simulink model "Motor_moddel"  (R2026a)
settings: Solver=VariableStepAuto
values from neighbouring files (symbols this model uses):
  B = 0.15    [Motor_model_param.m]
  gear = 9.68    [Motor_model_param.m]
  Kp = 0.05    [Motor_model_param.m]    (also in Vel_controller.m = 0.136458313659)
  wrad = 0.03    [Motor_model_param.m]
settings Model: Creator=mariu  LastModifiedBy=mariu

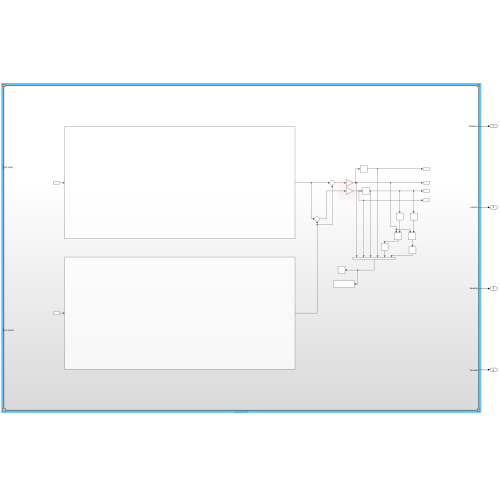
[thumbnail: Simulink's stored preview of the top-level diagram]
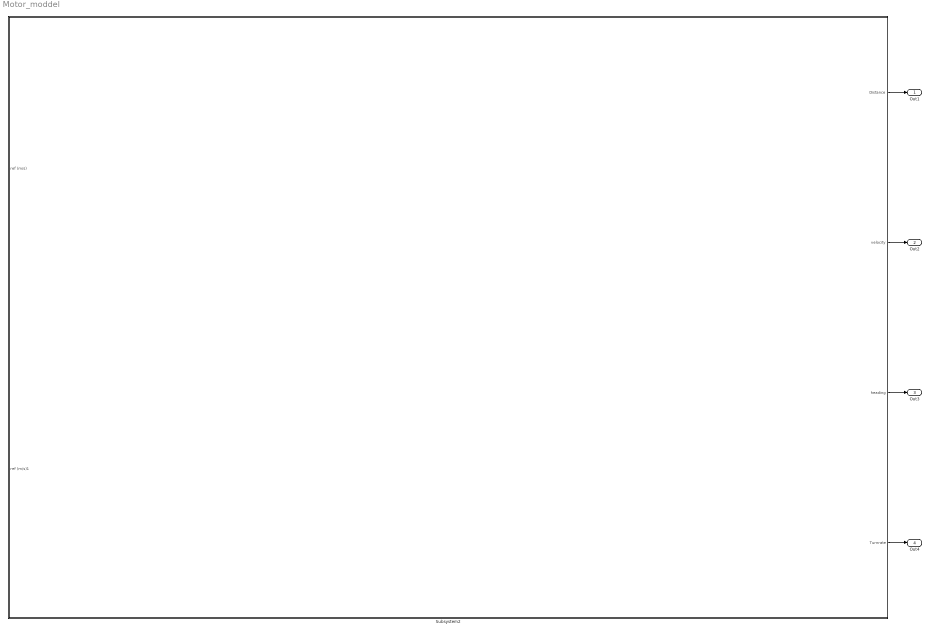
== system Motor_moddel ==
  Subsystem2 : Subsystem
  Out1 : Outport
  Out2 : Outport  Port=2
  Out3 : Outport  Port=3
  Out4 : Outport  Port=4
  wires:
  Subsystem2/1(Distance) -> Out1/1
  Subsystem2/2(velocity) -> Out2/1
  Subsystem2/3(heading) -> Out3/1
  Subsystem2/4(Turnrate) -> Out4/1

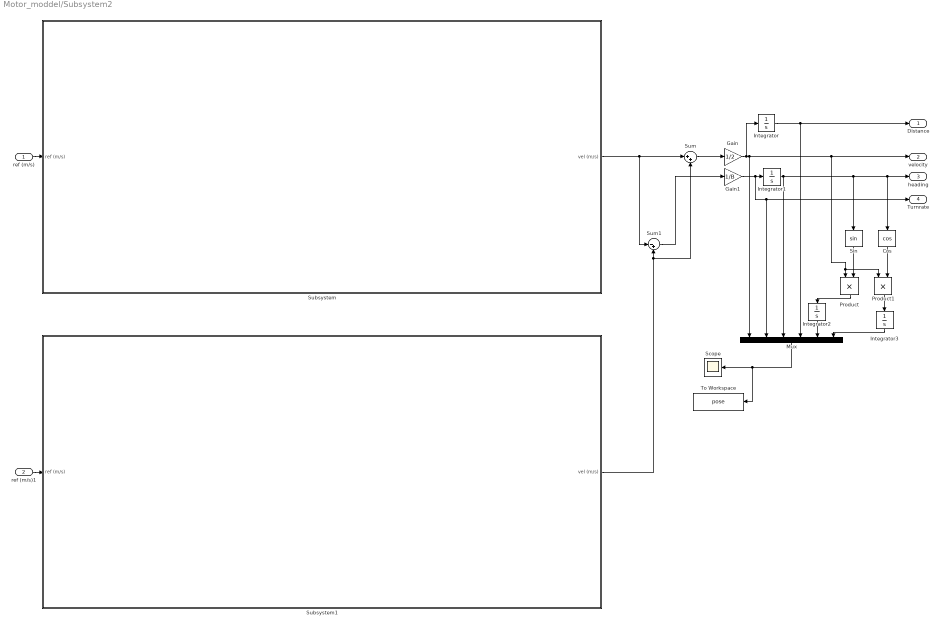
== system Motor_moddel/Subsystem2 ==
  ref (m/s) : Inport
  ref (m/s)1 : Inport  Port=2
  Cos : Trigonometry  Operator=cos
  Gain : Gain  Gain=1/2
  Gain1 : Gain  Gain=1/B
  Integrator{,1..3} (4 alike) : Integrator
  Mux : Mux  Inputs=6
  Product : Product
  Product1 : Product
  Scope : Scope
  Sin : Trigonometry
  Subsystem : Subsystem
  Subsystem1 : Subsystem
  Sum : Sum  Inputs=|++
  Sum1 : Sum  Inputs=|-+
  To Workspace : ToWorkspace  VariableName=pose  SaveFormat=Timeseries  SampleTime=-1
  Distance : Outport
  velocity : Outport  Port=2
  heading : Outport  Port=3
  Turnrate : Outport  Port=4
  wires:
  Integrator1/1 -> Mux/3, Sin/1, heading/1, Cos/1
  Subsystem/1(vel (m/s)) -> Sum1/1, Sum/1
  Gain/1 -> Mux/1, velocity/1, Product1/1, Product/1, Integrator/1
  Gain1/1 -> Turnrate/1, Mux/2, Integrator1/1
  Integrator3/1 -> Mux/6
  Subsystem1/1(vel (m/s)) -> Sum/2, Sum1/2
  Product1/1 -> Integrator3/1
  Mux/1 -> To Workspace/1, Scope/1
  Sum/1 -> Gain/1
  Integrator/1 -> Distance/1, Mux/4
  Sin/1 -> Product/2
  Integrator2/1 -> Mux/5
  Sum1/1 -> Gain1/1
  Cos/1 -> Product1/2
  Product/1 -> Integrator2/1
  ref (m/s)1/1 -> Subsystem1/1(ref (m/s))
  ref (m/s)/1 -> Subsystem/1(ref (m/s))

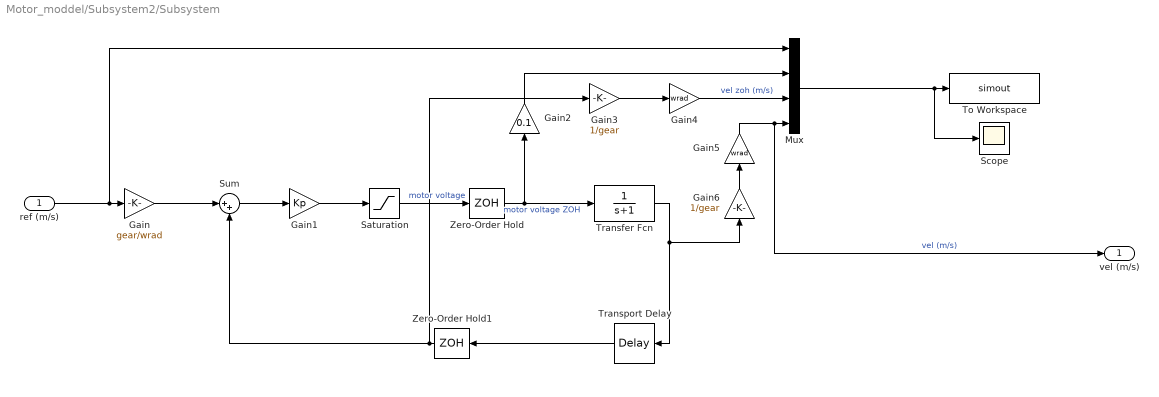
== system Motor_moddel/Subsystem2/Subsystem ==
  ref (m/s) : Inport
  Gain : Gain  Gain=gear/wrad
  Gain1 : Gain  Gain=Kp
  Gain2 : Gain  Gain=0.1
  Gain3 : Gain  Gain=1/gear
  Gain4 : Gain  Gain=wrad
  Gain5 : Gain  Gain=wrad
  Gain6 : Gain  Gain=1/gear
  Mux : Mux
  Saturation : Saturate
  Scope : Scope
  Sum : Sum  Inputs=|++
  To Workspace : ToWorkspace  VariableName=simout  SaveFormat=Timeseries  SampleTime=-1
  Transfer Fcn : TransferFcn  Denominator=[1 1]
  Transport Delay : TransportDelay  DelayTime=0.01
  Zero-Order Hold : ZeroOrderHold  SampleTime=-1
  Zero-Order Hold1 : ZeroOrderHold  SampleTime=-1
  vel (m/s) : Outport
  wires:
  Gain5/1 -> vel (m/s)/1, Mux/4  "vel (m/s)"
  Zero-Order Hold/1 -> Transfer Fcn/1, Gain2/1  "motor voltage ZOH"
  Gain4/1 -> Mux/3  "vel zoh (m/s)"
  Mux/1 -> Scope/1, To Workspace/1
  Gain6/1 -> Gain5/1
  Gain1/1 -> Saturation/1
  Gain2/1 -> Mux/2
  Transfer Fcn/1 -> Gain6/1, Transport Delay/1
  Gain3/1 -> Gain4/1
  Zero-Order Hold1/1 -> Gain3/1, Sum/2
  ref (m/s)/1 -> Mux/1, Gain/1
  Transport Delay/1 -> Zero-Order Hold1/1
  Saturation/1 -> Zero-Order Hold/1  "motor voltage"
  Gain/1 -> Sum/1
  Sum/1 -> Gain1/1

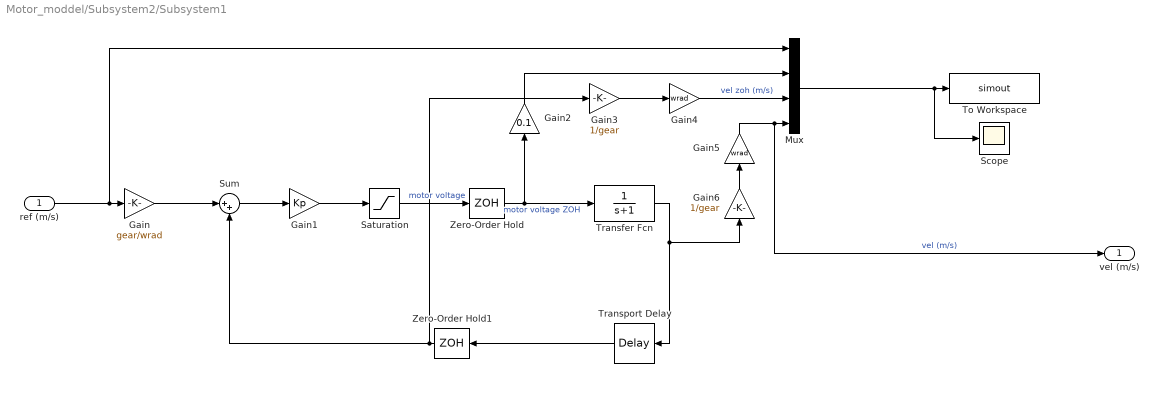
== system Motor_moddel/Subsystem2/Subsystem1 ==
  ref (m/s) : Inport
  Gain : Gain  Gain=gear/wrad
  Gain1 : Gain  Gain=Kp
  Gain2 : Gain  Gain=0.1
  Gain3 : Gain  Gain=1/gear
  Gain4 : Gain  Gain=wrad
  Gain5 : Gain  Gain=wrad
  Gain6 : Gain  Gain=1/gear
  Mux : Mux
  Saturation : Saturate
  Scope : Scope
  Sum : Sum  Inputs=|++
  To Workspace : ToWorkspace  VariableName=simout  SaveFormat=Timeseries  SampleTime=-1
  Transfer Fcn : TransferFcn  Denominator=[1 1]
  Transport Delay : TransportDelay  DelayTime=0.01
  Zero-Order Hold : ZeroOrderHold  SampleTime=-1
  Zero-Order Hold1 : ZeroOrderHold  SampleTime=-1
  vel (m/s) : Outport
  wires:
  Gain5/1 -> vel (m/s)/1, Mux/4  "vel (m/s)"
  Zero-Order Hold/1 -> Transfer Fcn/1, Gain2/1  "motor voltage ZOH"
  Gain4/1 -> Mux/3  "vel zoh (m/s)"
  Mux/1 -> Scope/1, To Workspace/1
  Gain6/1 -> Gain5/1
  Gain1/1 -> Saturation/1
  Gain2/1 -> Mux/2
  Transfer Fcn/1 -> Gain6/1, Transport Delay/1
  Gain3/1 -> Gain4/1
  Zero-Order Hold1/1 -> Gain3/1, Sum/2
  ref (m/s)/1 -> Mux/1, Gain/1
  Transport Delay/1 -> Zero-Order Hold1/1
  Saturation/1 -> Zero-Order Hold/1  "motor voltage"
  Gain/1 -> Sum/1
  Sum/1 -> Gain1/1
